simulink model "first_order_diff"  (R2022a)
settings: Solver=VariableStepAuto  StartTime=0.0  StopTime=10.0  RelTol=1e-3
settings Model: Creator=Home computer  LastModifiedBy=Home computer

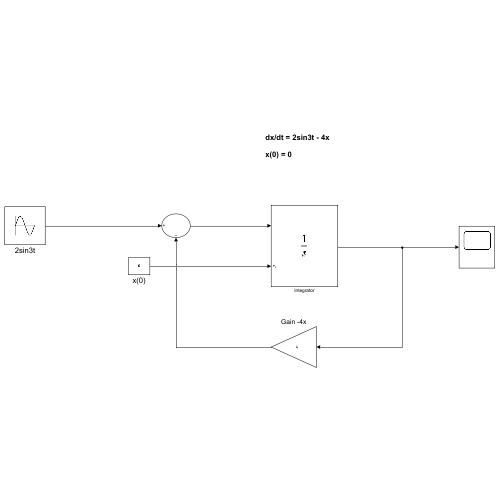
[thumbnail: Simulink's stored preview of the top-level diagram]
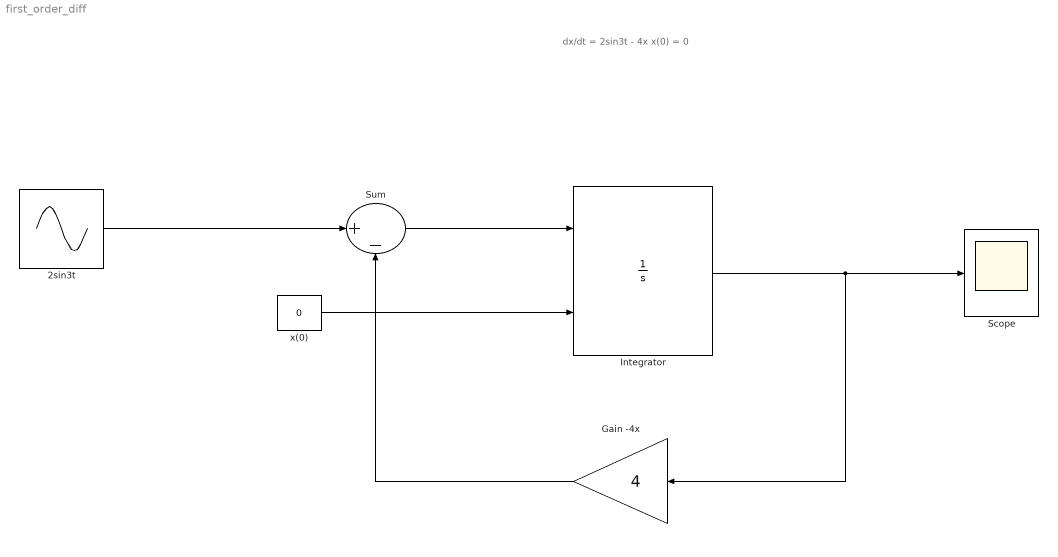
== system first_order_diff ==
  note: dx/dt = 2sin3t - 4x
      |
      | x(0) = 0
  2sin3t : Sin  Amplitude=2  Frequency=3  SampleTime=0
  Gain -4x : Gain  Gain=4
  Integrator : Integrator  InitialConditionSource=external
  Scope : Scope
  Sum : Sum  Inputs=|+-
  x(0) : Constant  Value=0
  wires:
  Integrator/1 -> Scope/1, Gain -4x/1
  Gain -4x/1 -> Sum/2
  Sum/1 -> Integrator/1
  2sin3t/1 -> Sum/1
  x(0)/1 -> Integrator/2
